simulink model "DDK_DCSUV_50ms"  (R2023b)
settings: Solver=FixedStepAuto  StartTime=0.0  StopTime=inf  FixedStep=0.001  RelTol=1e-3
InitFcn:
  | % 添加Python模块路径
  | py.sys.path().insert(int32(0), 'D:\YRJ_Workspace\DDK-python\MPC');
libraries: Solver_SF x1
settings Model: Creator=no_en  LastModifiedBy=Admin
settings SolverCC: AlgebraicLoopSolver=TrustRegion
settings DataIOCC: SaveState=on  ReturnWorkspaceOutputs=off
settings DebuggingCC: UnconnectedInputMsg=warning  UnconnectedOutputMsg=warning  UnconnectedLineMsg=warning  ArithmeticOperatorsInVariantConditions=warning
settings ModelReferenceCC: EnableRefExpFcnMdlSchedulingChecks=on
settings SFSimCC: SimUseLocalCustomCode=off  CustomCodeUndefinedFunction=UseInterfaceOnly
settings RTWCC: RTWUseLocalCustomCode=off  DLArmComputeVersion=19.05

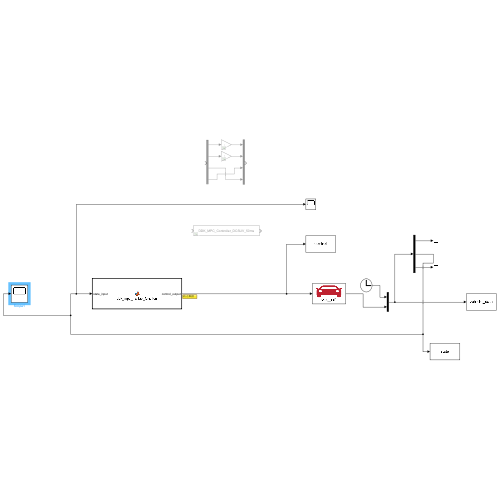
[thumbnail: Simulink's stored preview of the top-level diagram]
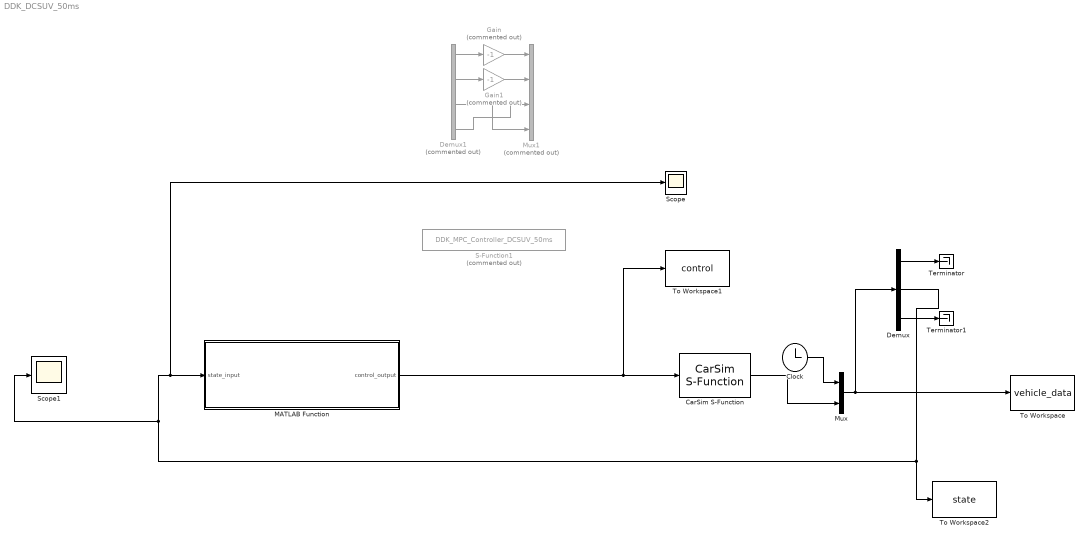
== system DDK_DCSUV_50ms ==
  CarSim S-Function : Solver_SF/CarSim S-Function  Priority=1  SIMFILE=simfile.sim  Run_RTs=off  vs_state_ind=Run  StopMode_ind=Vehicle Model
  Clock : Clock
  Demux : Demux  Outputs=[1 6 7]
  Demux1 : Demux  Commented=on
  Gain : Gain  Commented=on  Gain=-1
  Gain1 : Gain  Commented=on  Gain=-1
  MATLAB Function : MATLAB Function  TreatAsAtomicUnit=on
  Mux : Mux  Inputs=2
  Mux1 : Mux  Commented=on
  S-Function1 : S-Function  Commented=on  FunctionName=DDK_MPC_Controller_DCSUV_50ms  SFunctionDeploymentMode=off  EnableBusSupport=off
  Scope : Scope
  Scope1 : Scope
  Terminator : Terminator
  Terminator1 : Terminator
  To Workspace : ToWorkspace  VariableName=vehicle_data  SaveFormat=Timeseries  SampleTime=0.01
  To Workspace1 : ToWorkspace  VariableName=control  SaveFormat=Timeseries  SampleTime=0.01
  To Workspace2 : ToWorkspace  VariableName=state  SaveFormat=Timeseries  SampleTime=0.01
  wires:
  Clock/1 -> Mux/1
  CarSim S-Function/1 -> Mux/2
  Mux/1 -> Demux/1, To Workspace/1
  Demux/2 -> MATLAB Function/1(state_input), Scope/1, Scope1/1, To Workspace2/1
  MATLAB Function/1(control_output) -> To Workspace1/1, CarSim S-Function/1
  Demux/1 -> Terminator/1
  Demux/3 -> Terminator1/1
  Demux1/2 -> Gain1/1
  Gain/1 -> Mux1/1
  Gain1/1 -> Mux1/2
  Demux1/3 -> Mux1/4
  Demux1/1 -> Gain/1
  Demux1/4 -> Mux1/3

== matlab function DDK_DCSUV_50ms/MATLAB Function ==
  data: state_input input; control_output output
% MATLAB Function模块包装器
% 用于在Simulink中调用Python MPC控制器
%
% 使用方法：
% 1. 在Simulink中添加"MATLAB Function"块
% 2. 将此代码复制到MATLAB Function块中
% 3. 配置输入输出端口

function control_output = ddk_mpc_matlab_function(state_input)
%#codegen
% DDK-MPC控制器MATLAB Function包装器
%
% 输入:
%   state_input: [6x1] 车辆状态 [X, Y, Yaw(deg), vx(km/h), vy(km/h), yaw_rate(deg/s)]
%
% 输出:
%   control_output: [4x1] 控制信号 [steer_L1(deg), steer_R1(deg), throttle, brake]
%     对应原始MATLAB代码的 output = [steer_L1; steer_R1; throttle; brake]

% 显式声明输入输出大小（帮助代码生成器确定维度）
assert(isequal(size(state_input), [6, 1]), 'state_input must be 6x1');
control_output = zeros(4, 1);  % 预分配输出大小

% 声明Python函数为外部函数（不参与代码生成）
coder.extrinsic('py.ddk_mpc_sfunction.initialize_controller');
coder.extrinsic('py.ddk_mpc_sfunction.compute_control');
coder.extrinsic('py.ddk_mpc_sfunction.reset_controller');

% 持久变量（在仿真过程中保持状态）
persistent is_initialized;
persistent param_path;
persistent data_path;

% 初始化（第一次调用时）
if isempty(is_initialized)
    is_initialized = false;
    
    % 注意：运行前需在MATLAB命令窗口执行：
    % py.sys.path().insert(int32(0), 'D:\YRJ_Workspace\DDK-python\MPC');
    % py.eval('import ddk_mpc_sfunction');
    %
    % 设置路径（根据实际情况修改）
    param_path = 'D:\YRJ_Workspace\DDK-python\MPC\params_for_matlab_CarsimDClassSUV_2022_07_24_15_23.mat';
    data_path = 'D:\YRJ_Workspace\DDK-python\MPC\CarsimDClassSUVDatasets\Carsim_DClassSUV_test_0.mat';
    
    % 初始化Python控制器
    % 参数：param_path, data_path, Np=30, Nc=30, sample_interval=5
    py.ddk_mpc_sfunction.initialize_controller(param_path, data_path, 30, 30, 5);
    is_initialized = true;
end

% 调用Python MPC控制器
control_py = py.ddk_mpc_sfunction.compute_control(state_input);
control_output = double(control_py);
control_output = reshape(control_output(:), 4, 1);

% 安全检查
if numel(control_output) ~= 4
    control_output = zeros(4, 1);
end

end
